simulink model "model_FRT"  (R2022b)
settings: Solver=VariableStepAuto  StartTime=0.0  StopTime=30  RelTol=1e-3
values from neighbouring files (symbols this model uses):
  A_INV = [A_P                                        Z1                  Z3                   B_P ... (first row only)    [model_FRT_code.m]
  B_INV = [Z6 ... (first row only)    [model_FRT_code.m]
  C_f = (0.066*C_b)    (= 0.00220630670953)    [model_FRT_code.m]
  C_INV = [C_inv_w ... (first row only)    [model_FRT_code.m]
  D_INV = zeros(3,2)    [model_FRT_code.m]
  f_b = 50    [model_FRT_code.m]
  Kic = R_f/ti    (= 1.9044)    [model_FRT_code.m]
  Kiv = R_f/tiv    (= 0.19044)    [model_FRT_code.m]
  Kpc = L_f/ti    [model_FRT_code.m]
  Kpv = C_f*wm    [model_FRT_code.m]
  L_f = V_dc/(24*f_sw*delta_IL_max)    [model_FRT_code.m]
  L_g = 1*L_f    [model_FRT_code.m]
  mp = 0.01*50*2*pi/(S_b)    (= 6.28318530718e-07)    [model_FRT_code.m]
  nq = 2*V_m/(S_b)    [model_FRT_code.m]
  R_d = 0.2    [model_FRT_code.m]
  R_f = 0.008*Z_b    (= 0.00076176)    [model_FRT_code.m]
  R_g = 0.008*Z_b    (= 0.00076176)    [model_FRT_code.m]
  S_b = 5e6    (= 5000000)    [model_FRT_code.m]
  T_s = 100e-6    (= 0.0001)    [model_FRT_code.m]
  V_dc = 3*V_m    [model_FRT_code.m]
  V_m = sqrt(2/3)*V_b    [model_FRT_code.m]
  w_b = f_b*2*pi    (= 314.159265359)    [model_FRT_code.m]
  w_c = 0.1*w_b    (= 31.4159265359)    [model_FRT_code.m]
undefined symbols (not defined in the file or in its folder): G, K
libraries: slpidlib x8, spsabctodq0Lib x6, spsThreePhaseSeriesRLCBranchLib x4, spsPowerdq0InstantaneousLib x3, spsThreePhaseVIMeasurementLib x3, spsdq0toabcLib x3, spsGroundLib x2, spsDCVoltageSourceLib x1, spsPLL3phLib x1, spsPWMGenerator2LevelLib x1, spsPower3phPhasorLib x1, spsThreePhaseProgrammableVoltageSourceLib x1
(part 1 of 2)
settings Model: Creator=MSİ  LastModifiedBy=MSİ

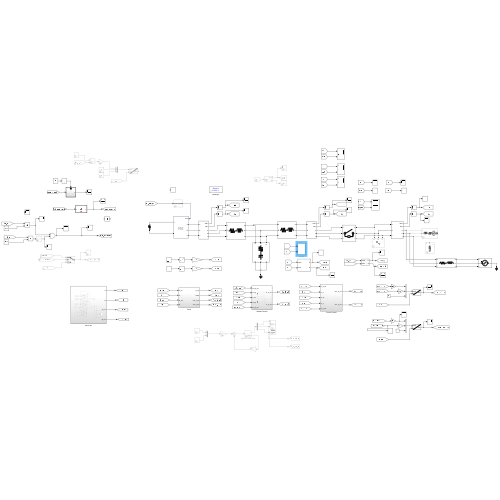
[thumbnail: Simulink's stored preview of the top-level diagram]
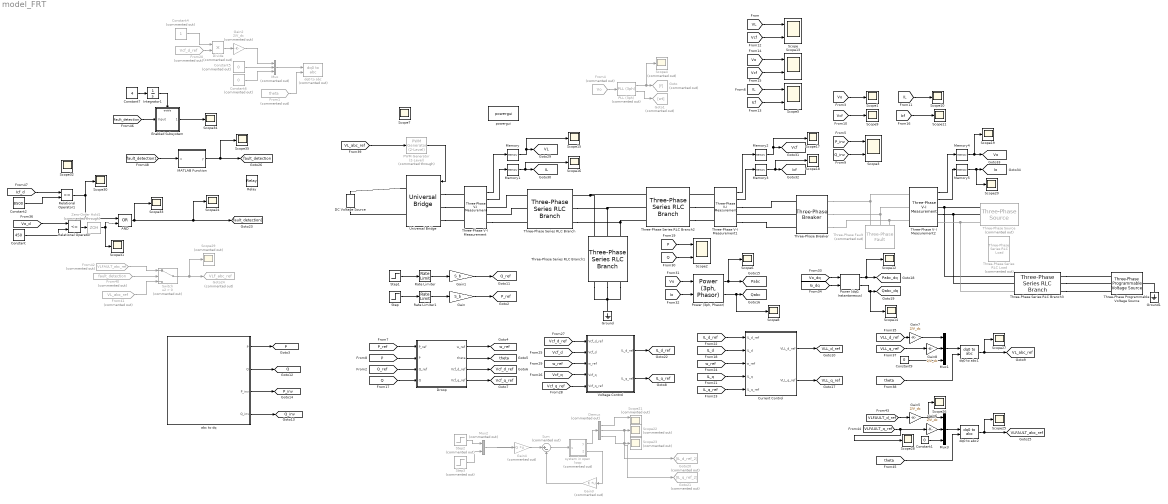
== system model_FRT ==
  AND : Logic  Operator=OR  IconShape=distinctive  AllPortsSameDT=off  OutDataTypeStr=boolean
  Constant : Constant  Value=450
  Constant1 : Constant  Value=0
  Constant2 : Constant  Value=8500
  Constant4 : Constant  Commented=on
  Constant5 : Constant  Commented=on  Value=0
  Constant6 : Constant  Commented=on  Value=0
  Constant7 : Constant  Value=4
  Constant9 : Constant  Value=0
  Current Control : Subsystem
  DC Voltage Source : spsDCVoltageSourceLib/DC Voltage Source  Amplitude=V_dc  Measurements=None
  Demux : Demux  Commented=on  Outputs=3
  Divide : Product  Commented=on  Inputs=**
  Droop : Subsystem
  Enabled Subsystem : Subsystem
  From1 : From  Commented=on  GotoTag=theta  TagVisibility=global
  From20 : From  Commented=on  GotoTag=Vcf_d_ref  TagVisibility=global
  From4 : From  Commented=on  GotoTag=Vo  TagVisibility=global
  From40 : From  Commented=on  GotoTag=fault_detection  TagVisibility=global
  From41 : From  Commented=on  GotoTag=VL_abc_ref  TagVisibility=global
  From42 : From  Commented=on  GotoTag=VLFAULT_abc_ref  TagVisibility=global
  Gain : Gain  Gain=S_b
  Gain1 : Gain  Gain=S_b
  Gain2 : Gain  Commented=on  Gain=2/V_dc
  Gain3 : Gain  Commented=on  Gain=K  Multiplication=Matrix(K*u)
  Gain4 : Gain  Commented=on  Gain=G  Multiplication=Matrix(K*u)
  Gain{5..8} (4 alike) : Gain  Gain=2/V_dc
  Goto : Goto  Commented=on  GotoTag=f
  Goto1 : Goto  Commented=on  GotoTag=wt
  Goto20 : Goto  Commented=on  GotoTag=IL_d_ref_2
  Goto21 : Goto  Commented=on  GotoTag=IL_q_ref_2
  Goto24 : Goto  Commented=on  GotoTag=VLF_abc_ref  TagVisibility=global
  Ground : spsGroundLib/Ground  LConnTagsString=a
  Ground1 : spsGroundLib/Ground  LConnTagsString=a
  Integrator1 : Integrator
  MATLAB Function : MATLAB Function  TreatAsAtomicUnit=on
  Memory{,1..5} (6 alike) : Memory
  Mux : Mux  Commented=on  Inputs=3
  Mux1 : Mux  Inputs=3
  Mux2 : Mux  Commented=on  Inputs=2
  Mux3 : Mux  Inputs=3
  PLL (3ph) : spsPLL3phLib/PLL (3ph)  Commented=on  Fmin=45  Par_Init=[0, 50]  ParK=[180, 3200, 1]  TcD=1e-4  MaxRateChangeFreq=12  FilterCutOffFreq=25  Ts=0  AGC=on
  PWM Generator (2-Level) : spsPWMGenerator2LevelLib/PWM Generator (2-Level)  Commented=through  ModulatorType=Three-phase bridge (6 pulses)  ModulatorMode=Unsynchronized  Fc=5000  Pc=-90  nF=5000/50  MinMax="[ -1  1 ]"  SamplingTechnique=Natural  ModulatingSignals=off  m=2/V_dc  Freq=50  Phase=0  Ts=0  ShowCarrierOutport=off
  "Power (3ph, Phasor)" : spsPower3phPhasorLib/Power (3ph, Phasor)
      settings: LibrarySourceBlock=|
      | sps_lib/Sensors and Measurements/Power
      | (3ph, Phasor)
  "Power (dq0, Instantaneous)" : spsPowerdq0InstantaneousLib/Power (dq0, Instantaneous)
      settings: LibrarySourceBlock=|
      | sps_lib/Sensors and Measurements/Power
      | (dq0, Instantaneous)
  Rate Limiter : RateLimiter  RisingSlewLimit=0.2  FallingSlewLimit=-0.2  SampleTimeMode=inherited
  Rate Limiter1 : RateLimiter  RisingSlewLimit=0.25  FallingSlewLimit=-0.1  SampleTimeMode=inherited
  Relational Operator : RelationalOperator  Operator=<=  OutDataTypeStr=boolean  RndMeth=Simplest  InputSameDT=off
  Relational Operator1 : RelationalOperator  OutDataTypeStr=boolean  RndMeth=Simplest  InputSameDT=off
  Relay : Relay
  Scope{,2..3,5,13} (5 alike) : Scope  NumInputPorts=2
  Scope{1,6..12,14..20,24..28,30..35} (26 alike) : Scope
  Scope21 : Scope  Commented=on  NumInputPorts=3
  Scope{4,22..23,29} (4 alike) : Scope  Commented=on
  Step : Step  Time=5  SampleTime=0
  Step1 : Step  Time=12  After=0.4  SampleTime=0
  Step2 : Step  Commented=on  After=100000  SampleTime=0
  Step3 : Step  Commented=on  Time=2  After=10000  SampleTime=0
  Sum : Sum  Commented=on  Inputs=|+-
  Switch : Switch  Commented=on  Criteria=u2 > Threshold  SaturateOnIntegerOverflow=off  InputSameDT=off
  Three-Phase Programmable Voltage Source : spsThreePhaseProgrammableVoltageSourceLib/Three-Phase Programmable Voltage Source  PositiveSequence="[690  0 50]"  VariationEntity=Phase  VariationType=Step  VariationTypeAlt=Step  VariationStep=10  VariationRate=2  VariationMagnitude=0.3  VariationFrequency=2  VariationTiming=[20 22]  VariationPhaseA=off  Amplitudes=[1 0.8 1.2 1.0]  TimeValues=[0 0.1 0.15 0.2]  HarmonicGeneration=off  HarmonicA=[3 0.2 -25 0]  HarmonicB=[2 0.15 35 2]  Timing="[0.05  3]"  BusType=swing  Pref=0  Qref=0  Qmin=-inf  Qmax=inf
  Three-Phase Series RLC Branch : spsThreePhaseSeriesRLCBranchLib/Three-Phase Series RLC Branch  LConnTagsString=A|B|C  RConnTagsString=A|B|C  BranchType=RL  Resistance=R_f  Inductance=L_f  Capacitance=1e-6  Measurements=None
  Three-Phase Series RLC Branch1 : spsThreePhaseSeriesRLCBranchLib/Three-Phase Series RLC Branch  LConnTagsString=A|B|C  RConnTagsString=A|B|C  BranchType=RC  Resistance=R_d  Inductance=1e-3  Capacitance=C_f  Measurements=None
  Three-Phase Series RLC Branch2 : spsThreePhaseSeriesRLCBranchLib/Three-Phase Series RLC Branch  LConnTagsString=A|B|C  RConnTagsString=A|B|C  BranchType=RL  Resistance=R_g  Inductance=L_g  Capacitance=1e-6  Measurements=None
  Three-Phase Series RLC Branch3 : spsThreePhaseSeriesRLCBranchLib/Three-Phase Series RLC Branch  LConnTagsString=A|B|C  RConnTagsString=A|B|C  BranchType=RL  Resistance=9.5e-4  Inductance=3e-5  Capacitance=1e-6  Measurements=None
  Three-Phase Series RLC Load : spsThreePhaseSeriesRLCLoadLib/Three-Phase Series RLC Load  Commented=on  LConnTagsString=A|B|C  Configuration=Y (grounded)  NominalVoltage=V_b  Vabc=[1e3 1e3 1e3]  Vabcp=[1e3 1e3 1e3]  NominalFrequency=50  UnbalancedPower=off  ActivePower=1e6  InductivePower=0  CapacitivePower=0  Pabc=[10e3 9e3 11e3]  QLabc=[100 90 110]  QCabc=[100 90 110]  Pabcp=[10e3 9e3 11e3]  QLabcp=[100 90 110]  QCabcp=[100 90 110]  Measurements=None  LoadType=constant Z
  Three-Phase V-I Measurement : spsThreePhaseVIMeasurementLib/Three-Phase V-I Measurement  VoltageMeasurement=phase-to-ground  SetLabelV=off  LabelV=VL  Vpu=off  VpuLL=off  CurrentMeasurement=yes  SetLabelI=off  LabelI=IL  Ipu=off  Pbase=100e6  Vbase=500e3  OutputType=Complex  PhasorSimulation=off  PSBequivalent=0
  Three-Phase V-I Measurement1 : spsThreePhaseVIMeasurementLib/Three-Phase V-I Measurement  VoltageMeasurement=phase-to-ground  SetLabelV=off  LabelV=Vcf  Vpu=off  VpuLL=off  CurrentMeasurement=yes  SetLabelI=off  LabelI=Icf  Ipu=off  Pbase=100e6  Vbase=500e3  OutputType=Complex  PhasorSimulation=off  PSBequivalent=0
  Three-Phase V-I Measurement2 : spsThreePhaseVIMeasurementLib/Three-Phase V-I Measurement  VoltageMeasurement=phase-to-ground  SetLabelV=off  LabelV=Vo  Vpu=off  VpuLL=off  CurrentMeasurement=yes  SetLabelI=off  LabelI=Io  Ipu=off  Pbase=100e6  Vbase=500e3  OutputType=Complex  PhasorSimulation=off  PSBequivalent=0
  Three-Phase Breaker : spsThreePhaseBreakerLib/Three-Phase Breaker  InitialState=open  SwitchA=on  SwitchB=on  SwitchC=on  SwitchTimes=[1]  External=off  BreakerResistance=0.01/10  SnubberResistance=1e6  SnubberCapacitance=inf  Measurements=None
  Three-Phase Fault : spsThreePhaseFaultLib/Three-Phase Fault  Commented=on  InitialStates=0  FaultA=on  FaultB=on  FaultC=on  GroundFault=on  SwitchTimes="[16  16.2]"  External=off  SwitchStatus=NaN  FaultResistance=0.1  GroundResistance=0.01  SnubberResistance=1e6  SnubberCapacitance=inf  Measurements=None
  Three-Phase Source : spsThreePhaseSourceLib/Three-Phase Source  Commented=on  InternalConnection=Yg  VoltagePhases=off  Voltage=(690)*1  PhaseAngle=0  Voltage_phases=[25e3 25e3 25e3]/sqrt(3)  PhaseAngles_phases=[0 -120 +120]  Frequency=f_b  NonIdealSource=on  SpecifyImpedance=on  Resistance=0.8929  Inductance=16.58e-3  ShortCircuitLevel=S_b*10  BaseVoltage=V_b  XRratio=10  BusType=swing  Pref=1000000  Qref=1000000  Prefabc=[10e3, 10e3, 10e3]  Qrefabc=[0, 0, 0]  Qmin=-Inf  Qmax=Inf
  Universal Bridge : spsUniversalBridgeLib/Universal Bridge  Arms=3  SnubberResistance=1e5  SnubberCapacitance=inf  Device=Average-model based VSC  Ron=1e-3  Lon=0  ForwardVoltages="[  0  0  ]"  ForwardVoltage=0  GTOparameters=[ 10e-6 , 20e-6 ]  IGBTparameters=[ 1e-6 , 2e-6 ]  Measurements=Device voltages  Measurements_2=None  converterType=Rectifier
  Voltage Control : Subsystem
  Zero-Order Hold1 : ZeroOrderHold  Commented=through  SampleTime=4
  abc to dq : Subsystem
  dq0 to abc : spsdq0toabcLib/dq0 to abc  Commented=on  Alignment=90 degrees behind phase A axis
  dq0 to abc1 : spsdq0toabcLib/dq0 to abc  Alignment=90 degrees behind phase A axis
  dq0 to abc2 : spsdq0toabcLib/dq0 to abc  Alignment=90 degrees behind phase A axis
  powergui : spspowerguiLib/powergui  Priority=1  SimulationMode=Discrete  SampleTime=T_s  frequency=60  Iterations=50  frequencyindice=0  Pbase=100e6  ErrMax=1e-4  UnitsV=kV  UnitsW=MW  buscounter=0  FunctionMessages=off  echomessages=off  EnableUseOfTLC=off  CurrentSourceSwitches=off  DisableSnubberDevices=off  DisableRonSwitches=off  DisableVfSwitches=off  DisplayEquations=off  AutomaticDiscreteSolvers=off  SolverType=Tustin/Backward Euler (TBE)  Interpol=off  ExternalGateDelay=off  methode=off  Ts=100  x0status=blocks  SPID=on  SwTol=0  HookPort=off  NonlinearTolerance=1e-4  nMaxIteration=100  ContinueOnMaxIteration=off  RestoreLinks=warning  ResistiveCurrentMeasurement=off  Frange=[0:2:500]  Ylog=off  Xlog=on  ShowGrid=off  save=off  variable=ZData  structure=0  ZoomFFT=off  StartTime=0.0  cycles=1  DisplayStyle=1  fundamental=60  FreqAxis=off  MaxFrequency=1000  frequencyindicesteady=1  RmsSteady=1  display=off
  system in open loop : Subsystem  Commented=on
  tag scope: IL=global, IL_d_ref=global, IL_q_ref=global, Icf=global, Io=global, P=global, P_inv=global, P_ref=global, Pabc=global, Pabc_dq=global, Q=global, Q_inv=global, Q_ref=global, Qabc=global, Qabc_dq=global, VL=global, VLFAULT_abc_ref=global, VLL_d_ref=global, VLL_q_ref=global, VL_abc_ref=global, Vcf=global, Vcf_d_ref=global, Vcf_q_ref=global, Vo=global, fault_detection1=global, fault_detection=global, theta=global, w_ref=global
  wires:
  [VL] -> Scope/1
  [Vo] -> Scope1/1
  From4/1 -> PLL (3ph)/1
  PLL (3ph)/1 -> Scope4/1, Goto/1
  PLL (3ph)/2 -> Goto1/1
  Constant5/1 -> Mux/2
  Constant6/1 -> Mux/3
  PWM Generator (2-Level)/1 -> Universal Bridge/1
  [IL] -> Scope5/1
  Step/1 -> Rate Limiter1/1
  Gain/1 -> [P_ref]
  [Vcf] -> Scope/2
  [Icf] -> Scope5/2
  [Vo] -> Scope13/1
  [Vcf] -> Scope13/2
  Gain1/1 -> [Q_ref]
  Step1/1 -> Rate Limiter/1
  Gain2/1 -> Mux/1
  From20/1 -> Divide/2
  Divide/1 -> Gain2/1
  Constant4/1 -> Divide/1
  [Vcf] -> Scope9/1
  [IL] -> Scope10/1
  [Icf] -> Scope11/1
  Constant9/1 -> Mux1/3
  Mux1/1 -> dq0 to abc1/1
  [theta] -> dq0 to abc1/2
  dq0 to abc1/1 -> Scope27/1, [VL_abc_ref]
  [VLL_d_ref] -> Gain7/1
  Gain7/1 -> Mux1/1
  Gain8/1 -> Mux1/2
  [VLL_q_ref] -> Gain8/1
  Mux/1 -> dq0 to abc/1
  From1/1 -> dq0 to abc/2
  [VL_abc_ref] -> PWM Generator (2-Level)/1
  [P_ref] -> Droop/1(P_ref)
  [P] -> Droop/2(P)
  [Q_ref] -> Droop/3(Q_ref)
  [Q] -> Droop/4(Q)
  Droop/1(w_ref) -> [w_ref]
  Droop/2(theta) -> [theta]
  Droop/3(Vcf_d_ref) -> [Vcf_d_ref]
  Droop/4(Vcf_q_ref) -> [Vcf_q_ref]
  [Vcf_d_ref] -> Voltage Control/1(Vcf_d_ref)
  [Vcf_d] -> Voltage Control/2(Vcf_d)
  [Vcf_q] -> Voltage Control/4(Vcf_q)
  [Vcf_q_ref] -> Voltage Control/5(Vcf_q_ref)
  Voltage Control/1(IL_d_ref) -> [IL_d_ref]
  Voltage Control/2(IL_q_ref) -> [IL_q_ref]
  [IL_d_ref] -> Current Control/1(IL_d_ref)
  [IL_d] -> Current Control/2(IL_d)
  [w_ref] -> Current Control/3(w_ref)
  [IL_q] -> Current Control/4(IL_q)
  [IL_q_ref] -> Current Control/5(IL_q_ref)
  Current Control/1(VLL_d_ref) -> [VLL_d_ref]
  Current Control/2(VLL_q_ref) -> [VLL_q_ref]
  Memory/1 -> Scope15/1, [VL]
  Memory1/1 -> Scope16/1, [IL]
  Three-Phase V-I Measurement/1 -> Memory/1
  Three-Phase V-I Measurement/2 -> Memory1/1
  Memory3/1 -> Scope18/1, [Icf]
  Memory2/1 -> Scope17/1, [Vcf]
  Three-Phase V-I Measurement1/1 -> Memory2/1
  Three-Phase V-I Measurement1/2 -> Memory3/1
  Memory4/1 -> Scope19/1, [Vo]
  Memory5/1 -> Scope20/1, [Io]
  Three-Phase V-I Measurement2/1 -> Memory4/1
  Three-Phase V-I Measurement2/2 -> Memory5/1
  abc to dq/2(Q) -> [Q]
  abc to dq/1(P) -> [P]
  [P] -> Scope2/1
  [Q] -> Scope2/2
  abc to dq/3(P_inv) -> [P_inv]
  abc to dq/4(Q_inv) -> [Q_inv]
  [P_inv] -> Scope3/1
  [Q_inv] -> Scope3/2
  [Vo] -> "Power (3ph, Phasor)"/1
  [Io] -> "Power (3ph, Phasor)"/2
  "Power (3ph, Phasor)"/1 -> Scope6/1, [Pabc]
  "Power (3ph, Phasor)"/2 -> Scope8/1, [Qabc]
  [Vo_dq] -> "Power (dq0, Instantaneous)"/1
  [Io_dq] -> "Power (dq0, Instantaneous)"/2
  "Power (dq0, Instantaneous)"/1 -> Scope12/1, [Pabc_dq]
  "Power (dq0, Instantaneous)"/2 -> Scope14/1, [Qabc_dq]
  Rate Limiter/1 -> Gain1/1
  Rate Limiter1/1 -> Gain/1
  [w_ref] -> Voltage Control/3(w_ref)
  Step2/1 -> Mux2/1
  Step3/1 -> Mux2/2
  system in open loop/1(y) -> Demux/1
  Demux/1 -> Scope21/1
  Mux2/1 -> Gain4/1
  Sum/1 -> system in open loop/1(u)
  Demux/2 -> Goto20/1, Scope22/1
  Demux/3 -> Goto21/1, Scope23/1
  Gain4/1 -> Sum/1
  system in open loop/2(state) -> Gain3/1
  Gain3/1 -> Sum/2
  [Vo_d] -> Relational Operator/1
  Constant/1 -> Relational Operator/2
  From40/1 -> Switch/2
  From41/1 -> Switch/3
  Switch/1 -> Scope29/1, Goto24/1
  From42/1 -> Switch/1
  Gain6/1 -> Mux3/2
  [theta] -> dq0 to abc2/2
  [VLFAULT_q_ref] -> Scope28/1, Gain6/1
  Mux3/1 -> dq0 to abc2/1
  dq0 to abc2/1 -> Scope25/1, [VLFAULT_abc_ref]
  Gain5/1 -> Scope26/1, Mux3/1
  Constant1/1 -> Mux3/3
  [VLFAULT_d_ref] -> Gain5/1
  AND/1 -> Scope24/1, [fault_detection1], Scope33/1
  Relational Operator/1 -> Zero-Order Hold1/1
  Relational Operator1/1 -> AND/1, Scope30/1
  Zero-Order Hold1/1 -> AND/2, Scope31/1
  [fault_detection] -> Enabled Subsystem/1(Input)
  Enabled Subsystem/1(Output) -> Scope34/1
  Constant7/1 -> Integrator1/1
  Integrator1/1 -> Enabled Subsystem/Enable
  [Icf_d] -> Relational Operator1/1
  Constant2/1 -> Relational Operator1/2
  MATLAB Function/1(y) -> Scope35/1, [fault_detection]
  [fault_detection1] -> MATLAB Function/1(u)
  connections:
  Universal Bridge/RConn1 -- DC Voltage Source/RConn1
  DC Voltage Source/LConn1 -- Universal Bridge/RConn2
  Three-Phase Series RLC Branch1/LConn1 -- Three-Phase Series RLC Branch2/LConn1 -- Three-Phase Series RLC Branch/RConn1
  Three-Phase Series RLC Branch/RConn2 -- Three-Phase Series RLC Branch2/LConn2 -- Three-Phase Series RLC Branch1/LConn2
  Three-Phase Series RLC Branch/RConn3 -- Three-Phase Series RLC Branch2/LConn3 -- Three-Phase Series RLC Branch1/LConn3
  Three-Phase Series RLC Branch1/RConn1 -- Three-Phase Series RLC Branch1/RConn3 -- Ground/LConn1 -- Three-Phase Series RLC Branch1/RConn2
  Three-Phase Series RLC Branch/LConn1 -- Three-Phase V-I Measurement/RConn1
  Three-Phase Series RLC Branch/LConn2 -- Three-Phase V-I Measurement/RConn2
  Universal Bridge/LConn1 -- Three-Phase V-I Measurement/LConn1
  Universal Bridge/LConn2 -- Three-Phase V-I Measurement/LConn2
  Universal Bridge/LConn3 -- Three-Phase V-I Measurement/LConn3
  Three-Phase V-I Measurement/RConn3 -- Three-Phase Series RLC Branch/LConn3
  Ground1/LConn1 -- Three-Phase Programmable Voltage Source/LConn1
  Three-Phase Fault/LConn1 -- Three-Phase V-I Measurement2/LConn1 -- Three-Phase Breaker/RConn1
  Three-Phase Fault/LConn2 -- Three-Phase V-I Measurement2/LConn2 -- Three-Phase Breaker/RConn2
  Three-Phase Fault/LConn3 -- Three-Phase V-I Measurement2/LConn3 -- Three-Phase Breaker/RConn3
  Three-Phase Series RLC Branch3/RConn1 -- Three-Phase Programmable Voltage Source/RConn1
  Three-Phase Series RLC Branch3/RConn2 -- Three-Phase Programmable Voltage Source/RConn2
  Three-Phase Series RLC Branch3/RConn3 -- Three-Phase Programmable Voltage Source/RConn3
  Three-Phase V-I Measurement2/RConn1 -- Three-Phase Series RLC Branch3/LConn1 -- Three-Phase Source/RConn1
  Three-Phase V-I Measurement2/RConn2 -- Three-Phase Series RLC Branch3/LConn2 -- Three-Phase Source/RConn2
  Three-Phase Source/RConn3 -- Three-Phase Series RLC Branch3/LConn3 -- Three-Phase V-I Measurement2/RConn3
  Three-Phase V-I Measurement1/LConn1 -- Three-Phase Series RLC Branch2/RConn1
  Three-Phase Series RLC Branch2/RConn2 -- Three-Phase V-I Measurement1/LConn2
  Three-Phase Series RLC Branch2/RConn3 -- Three-Phase V-I Measurement1/LConn3
  Three-Phase V-I Measurement1/RConn1 -- Three-Phase Breaker/LConn1
  Three-Phase Breaker/LConn2 -- Three-Phase V-I Measurement1/RConn2
  Three-Phase V-I Measurement1/RConn3 -- Three-Phase Breaker/LConn3

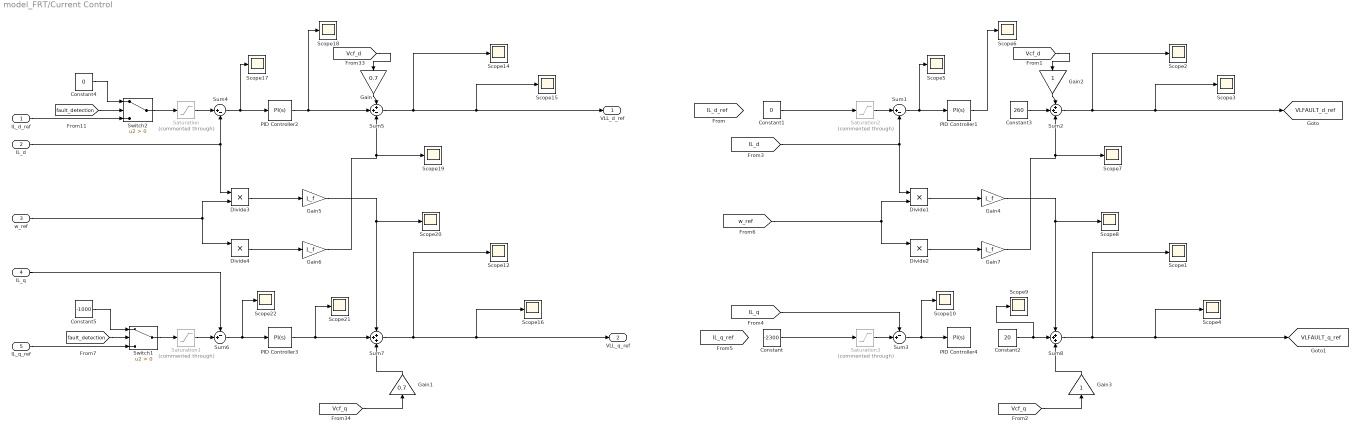
== system model_FRT/Current Control ==
  IL_d_ref : Inport
  IL_d : Inport  Port=2
  w_ref : Inport  Port=3
  IL_q : Inport  Port=4
  IL_q_ref : Inport  Port=5
  Constant : Constant  Value=-2300
  Constant1 : Constant  Value=0
  Constant2 : Constant  Value=20
  Constant3 : Constant  Value=260
  Constant4 : Constant  Value=0
  Constant5 : Constant  Value=-1000
  Divide{1..4} (4 alike) : Product  Inputs=**
  Gain : Gain  Gain=0.7
  Gain1 : Gain  Gain=0.7
  Gain2 : Gain
  Gain3 : Gain
  Gain{4..7} (4 alike) : Gain  Gain=L_f
  PID Controller1 : slpidlib/PID Controller  Controller=PI  Form=Parallel  TimeDomain=Continuous-time  UseExternalTs=off  SampleTime=-1  IntegratorMethod=Forward Euler  FilterMethod=Forward Euler  ControllerParametersSource=internal  P=Kpc  I=Kic  UseKiTs=off  D=0  N=100  UseFilter=on  TunerSelectOption=Transfer Function Based (PID Tuner App)  InitialConditionSource=internal  InitialConditionForIntegrator=0  InitialConditionForFilter=0  DifferentiatorICPrevScaledInput=0  ExternalReset=none  TrackingMode=off  Kt=1  LimitOutput=off  SatLimitsSource=internal  UpperSaturationLimit=60  LowerSaturationLimit=-60  LinearizeAsGain=on  AntiWindupMode=none  Kb=1  LimitIntegrator=off  UpperIntegratorSaturationLimit=inf  LowerIntegratorSaturationLimit=-inf  POutMin=[]  POutMax=[]  IOutMin=[]  IOutMax=[]  DOutMin=[]  DOutMax=[]  NOutMin=[]  NOutMax=[]  SumOutMin=[]  SumOutMax=[]  SaturationOutMin=[]  SaturationOutMax=[]  PParamMin=[]  PParamMax=[]  IParamMin=[]  IParamMax=[]  DParamMin=[]  DParamMax=[]  NParamMin=[]  NParamMax=[]  KbParamMin=[]  KbParamMax=[]  KtParamMin=[]  KtParamMax=[]  KbOutMin=[]  KbOutMax=[]  KtOutMin=[]  KtOutMax=[]  IntegratorOutMin=[]  IntegratorOutMax=[]  FilterOutMin=[]  FilterOutMax=[]  SumI1OutMin=[]  SumI1OutMax=[]  SumI2OutMin=[]  SumI2OutMax=[]  SumI3OutMin=[]  SumI3OutMax=[]  SumI4OutMin=[]  SumI4OutMax=[]  SumDOutMin=[]  SumDOutMax=[]  DifferentiatorOutMin=[]  DifferentiatorOutMax=[]  FilterDiffOutCoefMin=[]  FilterDiffOutCoefMax=[]  ReciprocalOutMin=[]  ReciprocalOutMax=[]  SumDenOutMin=[]  SumDenOutMax=[]  SumNumOutMin=[]  SumNumOutMax=[]  DivideOutMin=[]  DivideOutMax=[]  UdiffTsProdOutMin=[]  UdiffTsProdOutMax=[]  NTsProdOutMin=[]  NTsProdOutMax=[]  UintegralTsProdOutMin=[]  UintegralTsProdOutMax=[]  UngainTsProdOutMin=[]  UngainTsProdOutMax=[]  ClampingZeroOutDataTypeStr=Inherit: Inherit via back propagation  ClampingZeroOutMin=[]  ClampingZeroOutMax=[]  FilterDenConstantOutDataTypeStr=Inherit: Inherit via back propagation  FilterDenConstantOutMin=[]  FilterDenConstantOutMax=[]  PCopyOutDataTypeStr=Inherit: Inherit via back propagation  PCopyOutMin=[]  PCopyOutMax=[]  NCopyOutDataTypeStr=Inherit: Inherit via back propagation  NCopyOutMin=[]  NCopyOutMax=[]  IntegratorContinuousStateAttributes=''  IntegratorStateMustResolveToSignalObject=off  IntegratorRTWStateStorageClass=Auto  FilterContinuousStateAttributes=''  FilterStateMustResolveToSignalObject=off  FilterRTWStateStorageClass=Auto  ParallelPVariant=InternalParameters  IdealPVariant=Disabled  IVariant=InternalParameters  DVariant=Disabled  IntegratorVariant=Continuous  SatVariant=Disabled  AWVariant=Passthrough  PCopyVariant=Disabled  TRVariant=Disabled  FdbkBlocksVariant=Forward  IdealPFdbkVariant=Disabled  SatFdbkVariant=Disabled  DerivativeFilterVariant=Disabled  NVariant=Disabled  NCopyVariant=Disabled_SignalSpec  FilterICVariant=Disabled  IntegratorICVariant=InternalICs  ExternalResetVariant=Disabled  TRSumVariant=Passthrough  SumFdbkVariant=Disabled  SumVariant=Sum_PI  TsampFilterVariant=InternalTs  TsampNgainVariant=Passthrough  TsampIntegralVariant=Passthrough  ExternalSaturationOutDataTypeStr=Inherit: Same as second input
  PID Controller2 : slpidlib/PID Controller  Controller=PI  Form=Parallel  TimeDomain=Continuous-time  UseExternalTs=off  SampleTime=-1  IntegratorMethod=Forward Euler  FilterMethod=Forward Euler  ControllerParametersSource=internal  P=Kpc  I=Kic  UseKiTs=off  D=0  N=100  UseFilter=on  TunerSelectOption=Transfer Function Based (PID Tuner App)  InitialConditionSource=internal  InitialConditionForIntegrator=0  InitialConditionForFilter=0  DifferentiatorICPrevScaledInput=0  ExternalReset=none  TrackingMode=off  Kt=1  LimitOutput=off  SatLimitsSource=internal  UpperSaturationLimit=60  LowerSaturationLimit=-60  LinearizeAsGain=on  AntiWindupMode=none  Kb=1  LimitIntegrator=off  UpperIntegratorSaturationLimit=inf  LowerIntegratorSaturationLimit=-inf  POutMin=[]  POutMax=[]  IOutMin=[]  IOutMax=[]  DOutMin=[]  DOutMax=[]  NOutMin=[]  NOutMax=[]  SumOutMin=[]  SumOutMax=[]  SaturationOutMin=[]  SaturationOutMax=[]  PParamMin=[]  PParamMax=[]  IParamMin=[]  IParamMax=[]  DParamMin=[]  DParamMax=[]  NParamMin=[]  NParamMax=[]  KbParamMin=[]  KbParamMax=[]  KtParamMin=[]  KtParamMax=[]  KbOutMin=[]  KbOutMax=[]  KtOutMin=[]  KtOutMax=[]  IntegratorOutMin=[]  IntegratorOutMax=[]  FilterOutMin=[]  FilterOutMax=[]  SumI1OutMin=[]  SumI1OutMax=[]  SumI2OutMin=[]  SumI2OutMax=[]  SumI3OutMin=[]  SumI3OutMax=[]  SumI4OutMin=[]  SumI4OutMax=[]  SumDOutMin=[]  SumDOutMax=[]  DifferentiatorOutMin=[]  DifferentiatorOutMax=[]  FilterDiffOutCoefMin=[]  FilterDiffOutCoefMax=[]  ReciprocalOutMin=[]  ReciprocalOutMax=[]  SumDenOutMin=[]  SumDenOutMax=[]  SumNumOutMin=[]  SumNumOutMax=[]  DivideOutMin=[]  DivideOutMax=[]  UdiffTsProdOutMin=[]  UdiffTsProdOutMax=[]  NTsProdOutMin=[]  NTsProdOutMax=[]  UintegralTsProdOutMin=[]  UintegralTsProdOutMax=[]  UngainTsProdOutMin=[]  UngainTsProdOutMax=[]  ClampingZeroOutDataTypeStr=Inherit: Inherit via back propagation  ClampingZeroOutMin=[]  ClampingZeroOutMax=[]  FilterDenConstantOutDataTypeStr=Inherit: Inherit via back propagation  FilterDenConstantOutMin=[]  FilterDenConstantOutMax=[]  PCopyOutDataTypeStr=Inherit: Inherit via back propagation  PCopyOutMin=[]  PCopyOutMax=[]  NCopyOutDataTypeStr=Inherit: Inherit via back propagation  NCopyOutMin=[]  NCopyOutMax=[]  IntegratorContinuousStateAttributes=''  IntegratorStateMustResolveToSignalObject=off  IntegratorRTWStateStorageClass=Auto  FilterContinuousStateAttributes=''  FilterStateMustResolveToSignalObject=off  FilterRTWStateStorageClass=Auto  ParallelPVariant=InternalParameters  IdealPVariant=Disabled  IVariant=InternalParameters  DVariant=Disabled  IntegratorVariant=Continuous  SatVariant=Disabled  AWVariant=Passthrough  PCopyVariant=Disabled  TRVariant=Disabled  FdbkBlocksVariant=Forward  IdealPFdbkVariant=Disabled  SatFdbkVariant=Disabled  DerivativeFilterVariant=Disabled  NVariant=Disabled  NCopyVariant=Disabled_SignalSpec  FilterICVariant=Disabled  IntegratorICVariant=InternalICs  ExternalResetVariant=Disabled  TRSumVariant=Passthrough  SumFdbkVariant=Disabled  SumVariant=Sum_PI  TsampFilterVariant=InternalTs  TsampNgainVariant=Passthrough  TsampIntegralVariant=Passthrough  ExternalSaturationOutDataTypeStr=Inherit: Same as second input
  PID Controller3 : slpidlib/PID Controller  Controller=PI  Form=Parallel  TimeDomain=Continuous-time  UseExternalTs=off  SampleTime=-1  IntegratorMethod=Forward Euler  FilterMethod=Forward Euler  ControllerParametersSource=internal  P=Kpc  I=Kic  UseKiTs=off  D=0  N=100  UseFilter=on  TunerSelectOption=Transfer Function Based (PID Tuner App)  InitialConditionSource=internal  InitialConditionForIntegrator=0  InitialConditionForFilter=0  DifferentiatorICPrevScaledInput=0  ExternalReset=none  TrackingMode=off  Kt=1  LimitOutput=off  SatLimitsSource=internal  UpperSaturationLimit=26  LowerSaturationLimit=-20  LinearizeAsGain=on  AntiWindupMode=none  Kb=1  LimitIntegrator=off  UpperIntegratorSaturationLimit=inf  LowerIntegratorSaturationLimit=-inf  POutMin=[]  POutMax=[]  IOutMin=[]  IOutMax=[]  DOutMin=[]  DOutMax=[]  NOutMin=[]  NOutMax=[]  SumOutMin=[]  SumOutMax=[]  SaturationOutMin=[]  SaturationOutMax=[]  PParamMin=[]  PParamMax=[]  IParamMin=[]  IParamMax=[]  DParamMin=[]  DParamMax=[]  NParamMin=[]  NParamMax=[]  KbParamMin=[]  KbParamMax=[]  KtParamMin=[]  KtParamMax=[]  KbOutMin=[]  KbOutMax=[]  KtOutMin=[]  KtOutMax=[]  IntegratorOutMin=[]  IntegratorOutMax=[]  FilterOutMin=[]  FilterOutMax=[]  SumI1OutMin=[]  SumI1OutMax=[]  SumI2OutMin=[]  SumI2OutMax=[]  SumI3OutMin=[]  SumI3OutMax=[]  SumI4OutMin=[]  SumI4OutMax=[]  SumDOutMin=[]  SumDOutMax=[]  DifferentiatorOutMin=[]  DifferentiatorOutMax=[]  FilterDiffOutCoefMin=[]  FilterDiffOutCoefMax=[]  ReciprocalOutMin=[]  ReciprocalOutMax=[]  SumDenOutMin=[]  SumDenOutMax=[]  SumNumOutMin=[]  SumNumOutMax=[]  DivideOutMin=[]  DivideOutMax=[]  UdiffTsProdOutMin=[]  UdiffTsProdOutMax=[]  NTsProdOutMin=[]  NTsProdOutMax=[]  UintegralTsProdOutMin=[]  UintegralTsProdOutMax=[]  UngainTsProdOutMin=[]  UngainTsProdOutMax=[]  ClampingZeroOutDataTypeStr=Inherit: Inherit via back propagation  ClampingZeroOutMin=[]  ClampingZeroOutMax=[]  FilterDenConstantOutDataTypeStr=Inherit: Inherit via back propagation  FilterDenConstantOutMin=[]  FilterDenConstantOutMax=[]  PCopyOutDataTypeStr=Inherit: Inherit via back propagation  PCopyOutMin=[]  PCopyOutMax=[]  NCopyOutDataTypeStr=Inherit: Inherit via back propagation  NCopyOutMin=[]  NCopyOutMax=[]  IntegratorContinuousStateAttributes=''  IntegratorStateMustResolveToSignalObject=off  IntegratorRTWStateStorageClass=Auto  FilterContinuousStateAttributes=''  FilterStateMustResolveToSignalObject=off  FilterRTWStateStorageClass=Auto  ParallelPVariant=InternalParameters  IdealPVariant=Disabled  IVariant=InternalParameters  DVariant=Disabled  IntegratorVariant=Continuous  SatVariant=Disabled  AWVariant=Passthrough  PCopyVariant=Disabled  TRVariant=Disabled  FdbkBlocksVariant=Forward  IdealPFdbkVariant=Disabled  SatFdbkVariant=Disabled  DerivativeFilterVariant=Disabled  NVariant=Disabled  NCopyVariant=Disabled_SignalSpec  FilterICVariant=Disabled  IntegratorICVariant=InternalICs  ExternalResetVariant=Disabled  TRSumVariant=Passthrough  SumFdbkVariant=Disabled  SumVariant=Sum_PI  TsampFilterVariant=InternalTs  TsampNgainVariant=Passthrough  TsampIntegralVariant=Passthrough  ExternalSaturationOutDataTypeStr=Inherit: Same as second input
  PID Controller4 : slpidlib/PID Controller  Controller=PI  Form=Parallel  TimeDomain=Continuous-time  UseExternalTs=off  SampleTime=-1  IntegratorMethod=Forward Euler  FilterMethod=Forward Euler  ControllerParametersSource=internal  P=Kpc  I=Kic  UseKiTs=off  D=0  N=100  UseFilter=on  TunerSelectOption=Transfer Function Based (PID Tuner App)  InitialConditionSource=internal  InitialConditionForIntegrator=0  InitialConditionForFilter=0  DifferentiatorICPrevScaledInput=0  ExternalReset=none  TrackingMode=off  Kt=1  LimitOutput=off  SatLimitsSource=internal  UpperSaturationLimit=26  LowerSaturationLimit=-20  LinearizeAsGain=on  AntiWindupMode=none  Kb=1  LimitIntegrator=off  UpperIntegratorSaturationLimit=inf  LowerIntegratorSaturationLimit=-inf  POutMin=[]  POutMax=[]  IOutMin=[]  IOutMax=[]  DOutMin=[]  DOutMax=[]  NOutMin=[]  NOutMax=[]  SumOutMin=[]  SumOutMax=[]  SaturationOutMin=[]  SaturationOutMax=[]  PParamMin=[]  PParamMax=[]  IParamMin=[]  IParamMax=[]  DParamMin=[]  DParamMax=[]  NParamMin=[]  NParamMax=[]  KbParamMin=[]  KbParamMax=[]  KtParamMin=[]  KtParamMax=[]  KbOutMin=[]  KbOutMax=[]  KtOutMin=[]  KtOutMax=[]  IntegratorOutMin=[]  IntegratorOutMax=[]  FilterOutMin=[]  FilterOutMax=[]  SumI1OutMin=[]  SumI1OutMax=[]  SumI2OutMin=[]  SumI2OutMax=[]  SumI3OutMin=[]  SumI3OutMax=[]  SumI4OutMin=[]  SumI4OutMax=[]  SumDOutMin=[]  SumDOutMax=[]  DifferentiatorOutMin=[]  DifferentiatorOutMax=[]  FilterDiffOutCoefMin=[]  FilterDiffOutCoefMax=[]  ReciprocalOutMin=[]  ReciprocalOutMax=[]  SumDenOutMin=[]  SumDenOutMax=[]  SumNumOutMin=[]  SumNumOutMax=[]  DivideOutMin=[]  DivideOutMax=[]  UdiffTsProdOutMin=[]  UdiffTsProdOutMax=[]  NTsProdOutMin=[]  NTsProdOutMax=[]  UintegralTsProdOutMin=[]  UintegralTsProdOutMax=[]  UngainTsProdOutMin=[]  UngainTsProdOutMax=[]  ClampingZeroOutDataTypeStr=Inherit: Inherit via back propagation  ClampingZeroOutMin=[]  ClampingZeroOutMax=[]  FilterDenConstantOutDataTypeStr=Inherit: Inherit via back propagation  FilterDenConstantOutMin=[]  FilterDenConstantOutMax=[]  PCopyOutDataTypeStr=Inherit: Inherit via back propagation  PCopyOutMin=[]  PCopyOutMax=[]  NCopyOutDataTypeStr=Inherit: Inherit via back propagation  NCopyOutMin=[]  NCopyOutMax=[]  IntegratorContinuousStateAttributes=''  IntegratorStateMustResolveToSignalObject=off  IntegratorRTWStateStorageClass=Auto  FilterContinuousStateAttributes=''  FilterStateMustResolveToSignalObject=off  FilterRTWStateStorageClass=Auto  ParallelPVariant=InternalParameters  IdealPVariant=Disabled  IVariant=InternalParameters  DVariant=Disabled  IntegratorVariant=Continuous  SatVariant=Disabled  AWVariant=Passthrough  PCopyVariant=Disabled  TRVariant=Disabled  FdbkBlocksVariant=Forward  IdealPFdbkVariant=Disabled  SatFdbkVariant=Disabled  DerivativeFilterVariant=Disabled  NVariant=Disabled  NCopyVariant=Disabled_SignalSpec  FilterICVariant=Disabled  IntegratorICVariant=InternalICs  ExternalResetVariant=Disabled  TRSumVariant=Passthrough  SumFdbkVariant=Disabled  SumVariant=Sum_PI  TsampFilterVariant=InternalTs  TsampNgainVariant=Passthrough  TsampIntegralVariant=Passthrough  ExternalSaturationOutDataTypeStr=Inherit: Same as second input
  Saturation : Saturate  Commented=through  UpperLimit=1.1*5500  LowerLimit=-1.1*5500
  Saturation1 : Saturate  Commented=through  UpperLimit=600  LowerLimit=-1.1*4500
  Saturation2 : Saturate  Commented=through  UpperLimit=1.1*5500  LowerLimit=-1.1*5500
  Saturation3 : Saturate  Commented=through  UpperLimit=600  LowerLimit=-1.1*4500
  Scope{1..10,12,14..22} (20 alike) : Scope
  Sum1 : Sum  Inputs=|+-
  Sum2 : Sum  Inputs=++-
  Sum3 : Sum  Inputs=-+|
  Sum4 : Sum  Inputs=|+-
  Sum5 : Sum  Inputs=++-
  Sum6 : Sum  Inputs=-+|
  Sum7 : Sum  Inputs=+++
  Sum8 : Sum  Inputs=+++
  Switch1 : Switch  Criteria=u2 > Threshold  SaturateOnIntegerOverflow=off  InputSameDT=off
  Switch2 : Switch  Criteria=u2 > Threshold  SaturateOnIntegerOverflow=off  InputSameDT=off
  VLL_d_ref : Outport
  VLL_q_ref : Outport  Port=2
  tag scope: VLFAULT_d_ref=global, VLFAULT_q_ref=global
  wires:
  Sum5/1 -> VLL_d_ref/1, Scope15/1, Scope14/1
  Gain6/1 -> Scope19/1, Sum5/3
  Sum4/1 -> Scope17/1, PID Controller2/1
  PID Controller2/1 -> Scope18/1, Sum5/2
  PID Controller3/1 -> Scope21/1, Sum7/2
  Sum7/1 -> VLL_q_ref/1, Scope16/1, Scope12/1
  [Vcf_d] -> Gain/1
  Gain5/1 -> Scope20/1, Sum7/1
  Sum6/1 -> Scope22/1, PID Controller3/1
  Divide4/1 -> Gain6/1
  [Vcf_q] -> Gain1/1
  Divide3/1 -> Gain5/1
  IL_d/1 -> Sum4/2, Divide3/1
  w_ref/1 -> Divide4/1, Divide3/2
  IL_q/1 -> Sum6/1
  Gain/1 -> Sum5/1
  Gain1/1 -> Sum7/3
  Saturation/1 -> Sum4/1
  Saturation1/1 -> Sum6/2
  Saturation2/1 -> Sum1/1
  Gain2/1 -> Sum2/1
  Gain3/1 -> Sum8/3
  Sum1/1 -> Scope5/1, PID Controller1/1
  [IL_q] -> Sum3/1
  Constant/1 -> Saturation3/1
  [w_ref] -> Divide1/2, Divide2/1
  [IL_d] -> Sum1/2, Divide1/1
  Constant1/1 -> Saturation2/1
  [Vcf_q] -> Gain3/1
  Gain4/1 -> Scope8/1, Sum8/1
  Sum3/1 -> Scope10/1, PID Controller4/1
  Sum8/1 -> [VLFAULT_q_ref], Scope4/1, Scope1/1
  Divide2/1 -> Gain7/1
  PID Controller1/1 -> Scope6/1
  [Vcf_d] -> Gain2/1
  Gain7/1 -> Scope7/1, Sum2/3
  Saturation3/1 -> Sum3/2
  Divide1/1 -> Gain4/1
  Sum2/1 -> [VLFAULT_d_ref], Scope3/1, Scope2/1
  Constant2/1 -> Scope9/1, Sum8/2
  Constant3/1 -> Sum2/2
  [fault_detection] -> Switch2/2
  Switch2/1 -> Saturation/1
  IL_d_ref/1 -> Switch2/3
  Constant4/1 -> Switch2/1
  [fault_detection] -> Switch1/2
  Switch1/1 -> Saturation1/1
  IL_q_ref/1 -> Switch1/3
  Constant5/1 -> Switch1/1

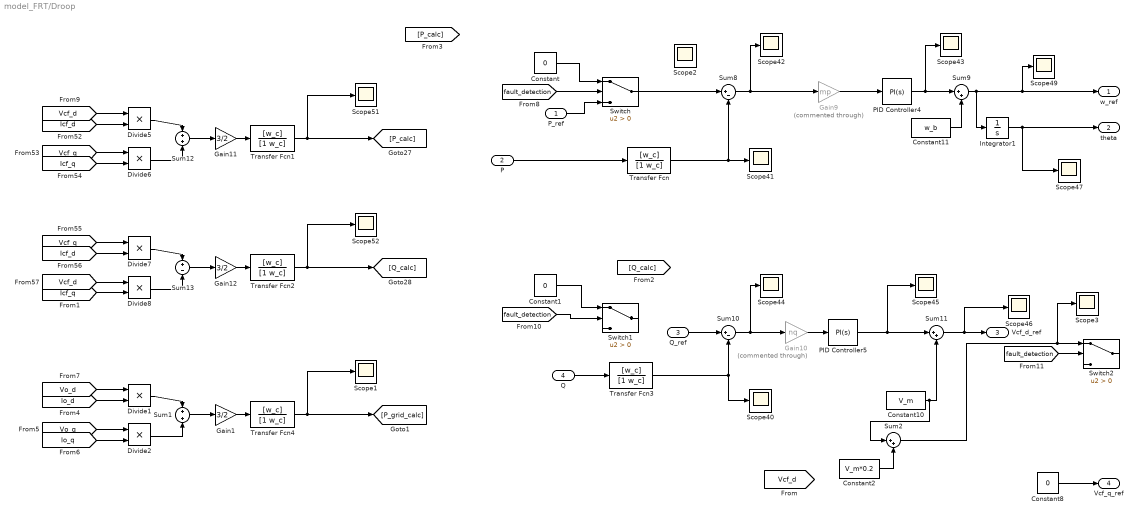
== system model_FRT/Droop ==
  P_ref : Inport
  P : Inport  Port=2
  Q_ref : Inport  Port=3
  Q : Inport  Port=4
  Constant : Constant  Value=0
  Constant1 : Constant  Value=0
  Constant10 : Constant  Value=V_m
  Constant11 : Constant  Value=w_b
  Constant2 : Constant  Value=V_m*0.2
  Constant8 : Constant  Value=0
  Divide{1..2,5..8} (6 alike) : Product  Inputs=**
  Gain1 : Gain  Gain=3/2
  Gain10 : Gain  Commented=through  Gain=nq
  Gain11 : Gain  Gain=3/2
  Gain12 : Gain  Gain=3/2
  Gain9 : Gain  Commented=through  Gain=mp
  Integrator1 : Integrator
  PID Controller4 : slpidlib/PID Controller  Controller=PI  Form=Parallel  TimeDomain=Continuous-time  UseExternalTs=off  SampleTime=-1  IntegratorMethod=Forward Euler  FilterMethod=Forward Euler  ControllerParametersSource=internal  P=mp  I=mp/10  UseKiTs=off  D=0  N=100  UseFilter=on  TunerSelectOption=Transfer Function Based (PID Tuner App)  InitialConditionSource=internal  InitialConditionForIntegrator=0  InitialConditionForFilter=0  DifferentiatorICPrevScaledInput=0  ExternalReset=none  TrackingMode=off  Kt=1  LimitOutput=off  SatLimitsSource=internal  UpperSaturationLimit=inf  LowerSaturationLimit=-inf  LinearizeAsGain=on  AntiWindupMode=none  Kb=1  LimitIntegrator=off  UpperIntegratorSaturationLimit=inf  LowerIntegratorSaturationLimit=-inf  POutMin=[]  POutMax=[]  IOutMin=[]  IOutMax=[]  DOutMin=[]  DOutMax=[]  NOutMin=[]  NOutMax=[]  SumOutMin=[]  SumOutMax=[]  SaturationOutMin=[]  SaturationOutMax=[]  PParamMin=[]  PParamMax=[]  IParamMin=[]  IParamMax=[]  DParamMin=[]  DParamMax=[]  NParamMin=[]  NParamMax=[]  KbParamMin=[]  KbParamMax=[]  KtParamMin=[]  KtParamMax=[]  KbOutMin=[]  KbOutMax=[]  KtOutMin=[]  KtOutMax=[]  IntegratorOutMin=[]  IntegratorOutMax=[]  FilterOutMin=[]  FilterOutMax=[]  SumI1OutMin=[]  SumI1OutMax=[]  SumI2OutMin=[]  SumI2OutMax=[]  SumI3OutMin=[]  SumI3OutMax=[]  SumI4OutMin=[]  SumI4OutMax=[]  SumDOutMin=[]  SumDOutMax=[]  DifferentiatorOutMin=[]  DifferentiatorOutMax=[]  FilterDiffOutCoefMin=[]  FilterDiffOutCoefMax=[]  ReciprocalOutMin=[]  ReciprocalOutMax=[]  SumDenOutMin=[]  SumDenOutMax=[]  SumNumOutMin=[]  SumNumOutMax=[]  DivideOutMin=[]  DivideOutMax=[]  UdiffTsProdOutMin=[]  UdiffTsProdOutMax=[]  NTsProdOutMin=[]  NTsProdOutMax=[]  UintegralTsProdOutMin=[]  UintegralTsProdOutMax=[]  UngainTsProdOutMin=[]  UngainTsProdOutMax=[]  ClampingZeroOutDataTypeStr=Inherit: Inherit via back propagation  ClampingZeroOutMin=[]  ClampingZeroOutMax=[]  FilterDenConstantOutDataTypeStr=Inherit: Inherit via back propagation  FilterDenConstantOutMin=[]  FilterDenConstantOutMax=[]  PCopyOutDataTypeStr=Inherit: Inherit via back propagation  PCopyOutMin=[]  PCopyOutMax=[]  NCopyOutDataTypeStr=Inherit: Inherit via back propagation  NCopyOutMin=[]  NCopyOutMax=[]  IntegratorContinuousStateAttributes=''  IntegratorStateMustResolveToSignalObject=off  IntegratorRTWStateStorageClass=Auto  FilterContinuousStateAttributes=''  FilterStateMustResolveToSignalObject=off  FilterRTWStateStorageClass=Auto  ParallelPVariant=InternalParameters  IdealPVariant=Disabled  IVariant=InternalParameters  DVariant=Disabled  IntegratorVariant=Continuous  SatVariant=Disabled  AWVariant=Passthrough  PCopyVariant=Disabled  TRVariant=Disabled  FdbkBlocksVariant=Forward  IdealPFdbkVariant=Disabled  SatFdbkVariant=Disabled  DerivativeFilterVariant=Disabled  NVariant=Disabled  NCopyVariant=Disabled_SignalSpec  FilterICVariant=Disabled  IntegratorICVariant=InternalICs  ExternalResetVariant=Disabled  TRSumVariant=Passthrough  SumFdbkVariant=Disabled  SumVariant=Sum_PI  TsampFilterVariant=InternalTs  TsampNgainVariant=Passthrough  TsampIntegralVariant=Passthrough  ExternalSaturationOutDataTypeStr=Inherit: Same as second input
  PID Controller5 : slpidlib/PID Controller  Controller=PI  Form=Parallel  TimeDomain=Continuous-time  UseExternalTs=off  SampleTime=-1  IntegratorMethod=Forward Euler  FilterMethod=Forward Euler  ControllerParametersSource=internal  P=nq  I=nq  UseKiTs=off  D=0  N=100  UseFilter=on  TunerSelectOption=Transfer Function Based (PID Tuner App)  InitialConditionSource=internal  InitialConditionForIntegrator=0  InitialConditionForFilter=0  DifferentiatorICPrevScaledInput=0  ExternalReset=none  TrackingMode=off  Kt=1  LimitOutput=off  SatLimitsSource=internal  UpperSaturationLimit=inf  LowerSaturationLimit=-inf  LinearizeAsGain=on  AntiWindupMode=none  Kb=1  LimitIntegrator=off  UpperIntegratorSaturationLimit=inf  LowerIntegratorSaturationLimit=-inf  POutMin=[]  POutMax=[]  IOutMin=[]  IOutMax=[]  DOutMin=[]  DOutMax=[]  NOutMin=[]  NOutMax=[]  SumOutMin=[]  SumOutMax=[]  SaturationOutMin=[]  SaturationOutMax=[]  PParamMin=[]  PParamMax=[]  IParamMin=[]  IParamMax=[]  DParamMin=[]  DParamMax=[]  NParamMin=[]  NParamMax=[]  KbParamMin=[]  KbParamMax=[]  KtParamMin=[]  KtParamMax=[]  KbOutMin=[]  KbOutMax=[]  KtOutMin=[]  KtOutMax=[]  IntegratorOutMin=[]  IntegratorOutMax=[]  FilterOutMin=[]  FilterOutMax=[]  SumI1OutMin=[]  SumI1OutMax=[]  SumI2OutMin=[]  SumI2OutMax=[]  SumI3OutMin=[]  SumI3OutMax=[]  SumI4OutMin=[]  SumI4OutMax=[]  SumDOutMin=[]  SumDOutMax=[]  DifferentiatorOutMin=[]  DifferentiatorOutMax=[]  FilterDiffOutCoefMin=[]  FilterDiffOutCoefMax=[]  ReciprocalOutMin=[]  ReciprocalOutMax=[]  SumDenOutMin=[]  SumDenOutMax=[]  SumNumOutMin=[]  SumNumOutMax=[]  DivideOutMin=[]  DivideOutMax=[]  UdiffTsProdOutMin=[]  UdiffTsProdOutMax=[]  NTsProdOutMin=[]  NTsProdOutMax=[]  UintegralTsProdOutMin=[]  UintegralTsProdOutMax=[]  UngainTsProdOutMin=[]  UngainTsProdOutMax=[]  ClampingZeroOutDataTypeStr=Inherit: Inherit via back propagation  ClampingZeroOutMin=[]  ClampingZeroOutMax=[]  FilterDenConstantOutDataTypeStr=Inherit: Inherit via back propagation  FilterDenConstantOutMin=[]  FilterDenConstantOutMax=[]  PCopyOutDataTypeStr=Inherit: Inherit via back propagation  PCopyOutMin=[]  PCopyOutMax=[]  NCopyOutDataTypeStr=Inherit: Inherit via back propagation  NCopyOutMin=[]  NCopyOutMax=[]  IntegratorContinuousStateAttributes=''  IntegratorStateMustResolveToSignalObject=off  IntegratorRTWStateStorageClass=Auto  FilterContinuousStateAttributes=''  FilterStateMustResolveToSignalObject=off  FilterRTWStateStorageClass=Auto  ParallelPVariant=InternalParameters  IdealPVariant=Disabled  IVariant=InternalParameters  DVariant=Disabled  IntegratorVariant=Continuous  SatVariant=Disabled  AWVariant=Passthrough  PCopyVariant=Disabled  TRVariant=Disabled  FdbkBlocksVariant=Forward  IdealPFdbkVariant=Disabled  SatFdbkVariant=Disabled  DerivativeFilterVariant=Disabled  NVariant=Disabled  NCopyVariant=Disabled_SignalSpec  FilterICVariant=Disabled  IntegratorICVariant=InternalICs  ExternalResetVariant=Disabled  TRSumVariant=Passthrough  SumFdbkVariant=Disabled  SumVariant=Sum_PI  TsampFilterVariant=InternalTs  TsampNgainVariant=Passthrough  TsampIntegralVariant=Passthrough  ExternalSaturationOutDataTypeStr=Inherit: Same as second input
  Scope{1..3,40..47,49,51..52} (14 alike) : Scope
  Sum1 : Sum  Inputs=+|+
  Sum10 : Sum  Inputs=|+-
  Sum11 : Sum  Inputs=|++
  Sum12 : Sum  Inputs=+|+
  Sum13 : Sum  Inputs=+|-
  Sum2 : Sum  Inputs=|++
  Sum8 : Sum  Inputs=|+-
  Sum9 : Sum  Inputs=|++
  Switch : Switch  Criteria=u2 > Threshold  SaturateOnIntegerOverflow=off  InputSameDT=off
  Switch1 : Switch  Criteria=u2 > Threshold  SaturateOnIntegerOverflow=off  InputSameDT=off
  Switch2 : Switch  Criteria=u2 > Threshold  SaturateOnIntegerOverflow=off  InputSameDT=off
  Transfer Fcn{,1..4} (5 alike) : TransferFcn  Numerator=[w_c]  Denominator=[1 w_c]
  w_ref : Outport
  theta : Outport  Port=2
  Vcf_d_ref : Outport  Port=3
  Vcf_q_ref : Outport  Port=4
  wires:
  Integrator1/1 -> theta/1, Scope47/1
  Constant8/1 -> Vcf_q_ref/1
  Sum9/1 -> Integrator1/1, w_ref/1, Scope49/1
  Sum10/1 -> Scope44/1, Gain10/1
  Gain9/1 -> PID Controller4/1
  Sum8/1 -> Scope42/1, Gain9/1
  PID Controller4/1 -> Scope43/1, Sum9/1
  Constant11/1 -> Sum9/2
  Constant10/1 -> Sum2/1, Sum11/2
  Gain10/1 -> PID Controller5/1
  Gain12/1 -> Transfer Fcn2/1
  Transfer Fcn1/1 -> Scope51/1, [P_calc]
  Transfer Fcn2/1 -> Scope52/1, [Q_calc]
  [Icf_d] -> Divide5/2
  Sum13/1 -> Gain12/1
  [Vcf_d] -> Divide8/1
  Divide5/1 -> Sum12/1
  [Vcf_q] -> Divide7/1
  [Icf_d] -> Divide7/2
  [Vcf_d] -> Divide5/1
  Divide8/1 -> Sum13/2
  [Vcf_q] -> Divide6/1
  [Icf_q] -> Divide6/2
  Gain11/1 -> Transfer Fcn1/1
  Sum12/1 -> Gain11/1
  Divide6/1 -> Sum12/2
  Divide7/1 -> Sum13/1
  [Icf_q] -> Divide8/2
  P/1 -> Transfer Fcn/1
  PID Controller5/1 -> Scope45/1, Sum11/1
  Q/1 -> Transfer Fcn3/1
  Transfer Fcn/1 -> Sum8/2, Scope41/1
  Transfer Fcn3/1 -> Scope40/1, Sum10/2
  Divide2/1 -> Sum1/2
  [Vo_q] -> Divide2/1
  Divide1/1 -> Sum1/1
  [Vo_d] -> Divide1/1
  Sum1/1 -> Gain1/1
  Transfer Fcn4/1 -> Scope1/1, [P_grid_calc]
  Gain1/1 -> Transfer Fcn4/1
  [Io_q] -> Divide2/2
  [Io_d] -> Divide1/2
  [fault_detection] -> Switch/2
  Constant/1 -> Switch/1
  [fault_detection] -> Switch1/2
  Constant1/1 -> Switch1/1
  [fault_detection] -> Switch2/2
  Sum2/1 -> Scope3/1, Switch2/1
  Constant2/1 -> Sum2/2
  Q_ref/1 -> Sum10/1
  Sum11/1 -> Scope46/1, Vcf_d_ref/1
  P_ref/1 -> Switch/3
  Switch/1 -> Sum8/1

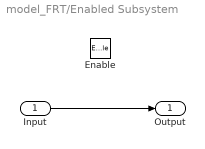
== system model_FRT/Enabled Subsystem ==
  Input : Inport
  Enable : EnablePort
  Output : Outport
  wires:
  Input/1 -> Output/1
